simulink model "PiFace_Modbus_task"  (Simulink 3.00)
libraries: logiclib x32

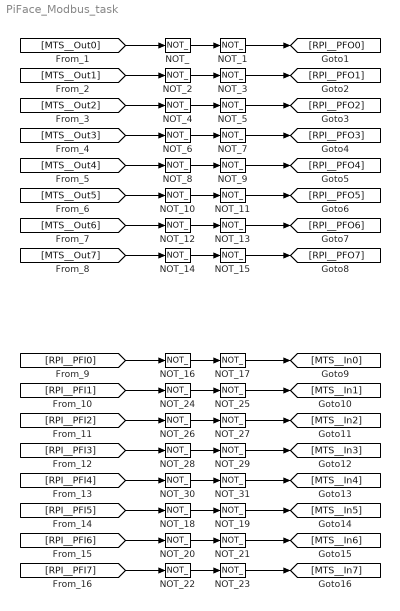
== system PiFace_Modbus_task ==
  NOT_{,1..31} (32 alike) : logiclib/NOT_
  wires:
  [MTS__Out0] -> NOT_/1
  [RPI__PFI1] -> NOT_24/1
  [RPI__PFI2] -> NOT_26/1
  [RPI__PFI3] -> NOT_28/1
  [RPI__PFI4] -> NOT_30/1
  [RPI__PFI5] -> NOT_18/1
  [RPI__PFI6] -> NOT_20/1
  [RPI__PFI7] -> NOT_22/1
  [MTS__Out1] -> NOT_2/1
  [MTS__Out2] -> NOT_4/1
  [MTS__Out3] -> NOT_6/1
  [MTS__Out4] -> NOT_8/1
  [MTS__Out5] -> NOT_10/1
  [MTS__Out6] -> NOT_12/1
  [MTS__Out7] -> NOT_14/1
  [RPI__PFI0] -> NOT_16/1
  NOT_/1 -> NOT_1/1
  NOT_1/1 -> [RPI__PFO0]
  NOT_10/1 -> NOT_11/1
  NOT_11/1 -> [RPI__PFO5]
  NOT_12/1 -> NOT_13/1
  NOT_13/1 -> [RPI__PFO6]
  NOT_14/1 -> NOT_15/1
  NOT_15/1 -> [RPI__PFO7]
  NOT_16/1 -> NOT_17/1
  NOT_17/1 -> [MTS__In0]
  NOT_18/1 -> NOT_19/1
  NOT_19/1 -> [MTS__In5]
  NOT_2/1 -> NOT_3/1
  NOT_20/1 -> NOT_21/1
  NOT_21/1 -> [MTS__In6]
  NOT_22/1 -> NOT_23/1
  NOT_23/1 -> [MTS__In7]
  NOT_24/1 -> NOT_25/1
  NOT_25/1 -> [MTS__In1]
  NOT_26/1 -> NOT_27/1
  NOT_27/1 -> [MTS__In2]
  NOT_28/1 -> NOT_29/1
  NOT_29/1 -> [MTS__In3]
  NOT_3/1 -> [RPI__PFO1]
  NOT_30/1 -> NOT_31/1
  NOT_31/1 -> [MTS__In4]
  NOT_4/1 -> NOT_5/1
  NOT_5/1 -> [RPI__PFO2]
  NOT_6/1 -> NOT_7/1
  NOT_7/1 -> [RPI__PFO3]
  NOT_8/1 -> NOT_9/1
  NOT_9/1 -> [RPI__PFO4]
